simulink subsystem "Subsystem_Driver_Cruise_BAv01"  (R2022b)
settings: Solver=VariableStepAuto  StartTime=0.0  StopTime=10.0  RelTol=1e-3
settings Model: Creator=giaco  LastModifiedBy=giaco

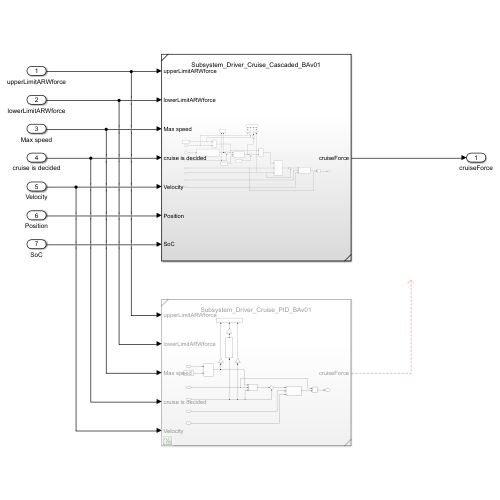
[thumbnail: Simulink's stored preview of the top-level diagram]
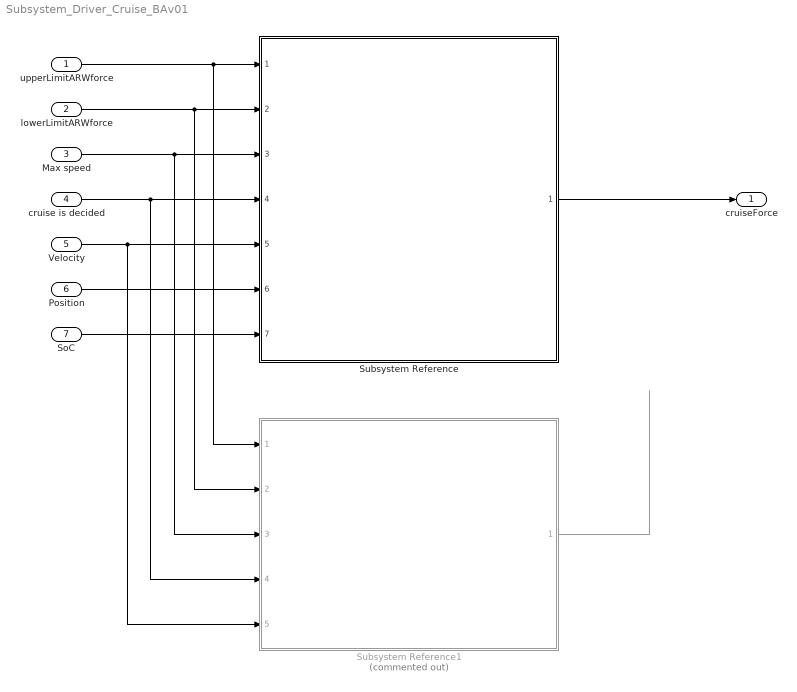
== system Subsystem_Driver_Cruise_BAv01 ==
  upperLimitARWforce : Inport
  lowerLimitARWforce : Inport  Port=2
  Max speed : Inport  Port=3
  cruise is decided : Inport  Port=4
  Velocity : Inport  Port=5
  Position : Inport  Port=6
  SoC : Inport  Port=7
  Subsystem Reference : Subsystem  ReferencedSubsystem=Subsystem_Driver_Cruise_Cascaded_BAv01
  Subsystem Reference1 : Subsystem  Commented=on  ReferencedSubsystem=Subsystem_Driver_Cruise_PID_BAv01
  cruiseForce : Outport
  wires:
  Max speed/1 -> Subsystem Reference1/3, Subsystem Reference/3
  Position/1 -> Subsystem Reference/6
  cruise is decided/1 -> Subsystem Reference1/4, Subsystem Reference/4
  SoC/1 -> Subsystem Reference/7
  Velocity/1 -> Subsystem Reference1/5, Subsystem Reference/5
  upperLimitARWforce/1 -> Subsystem Reference1/1, Subsystem Reference/1
  lowerLimitARWforce/1 -> Subsystem Reference1/2, Subsystem Reference/2
  Subsystem Reference/1 -> cruiseForce/1
  Subsystem Reference1/1 -> ?
